simulink model "sysgenImageDoubleBuffer"  (Simulink 7.7)
settings: Solver=VariableStepDiscrete  StartTime=0.0  StopTime=((c_rx_rows_2*c_rx_cols_2)*2+(320*10))+5000  RelTol=1e-3
PreLoadFcn:
  | sysgenImageDoubleBuffer_PreLoadFcn
StartFcn:
  | tic;
undefined symbols (not defined in the file or in its folder): c_rx_cols_1, c_rx_cols_2, c_rx_rows_1, c_rx_rows_2, dpost_1, dpost_2
libraries: xbsIndex_r4 x160, dspbuff3 x6, dspsigattribs x6, dspmtrx3 x6, vipsrcs x2, simulink x2, xbsCopyrightNotice_r4 x1
(part 1 of 3)
settings Model: Creator=arvinds  LastModifiedBy=wayneh

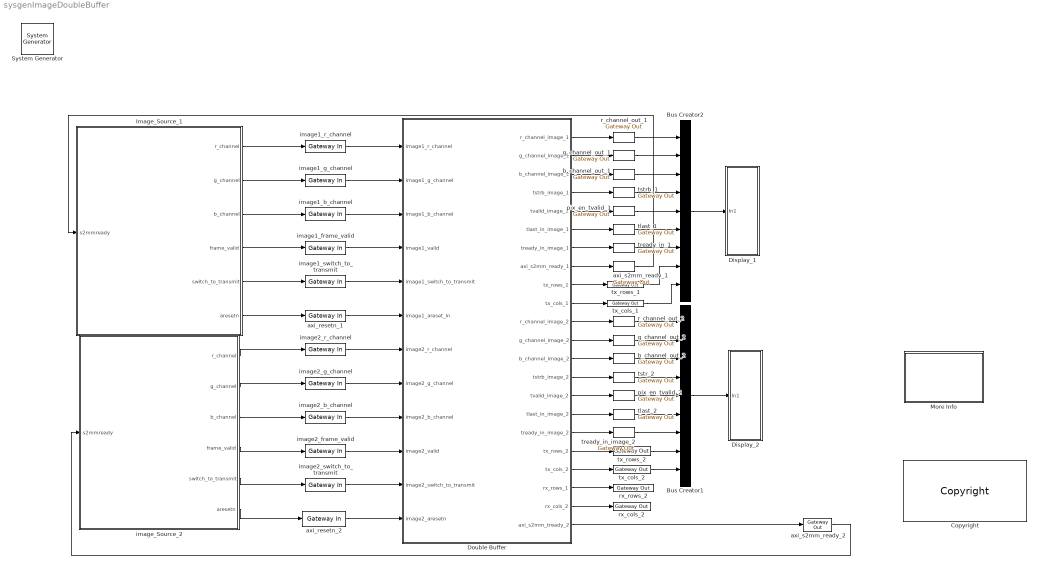
== system sysgenImageDoubleBuffer ==
  " System Generator" : xbsIndex_r4/ System Generator  Tag=genX  SystemSampleTime=-1  xilinxfamily=virtex6  part=xc6vlx240t  speed=-1  package=ff1156  synthesis_tool=XST  clock_wrapper=Clock Enables  directory=./netlist  proj_type=Project Navigator  Synth_file=XST Defaults  Impl_file=ISE Defaults  testbench=off  simulink_period=1  sysclk_period=10  dcm_input_clock_period=10  incr_netlist=off  trim_vbits=Everywhere in SubSystem  dbl_ovrd=According to Block Masks  core_generation=According to Block Masks  run_coregen=off  deprecated_control=off  eval_field=0  block_type=sysgen
      settings: block_version=12.3
  Bus Creator1 : BusCreator  Inputs=9
  Bus Creator2 : BusCreator  Inputs=9
  Copyright : xbsCopyrightNotice_r4/Copyright  copyrighttext="Copyright (c) 2011  by  Xilinx, Inc. All rights reserved.<br><br>This file contains proprietary, confidential information of Xilinx, Inc., is distributed under license from Xilinx, Inc., and may be used, copied and/or disclosed only pursuant to the terms of a valid license agreement with Xilinx, Inc. Xilinx hereby grants you a license to use this file solely for design, simulation, implementation and creation of design files limited to Xilinx devices or technologies. Use with non-Xilinx devices or technologies is expressly prohibited and immediately terminates your license unless covered by a separate agreement.<br><br>Xilinx is providing this design, code, or information \"as-is\" solely for use in developing programs and solutions for Xilinx devices, with no obligation on the part of Xilinx to provide support. By providing this design, code, or information as one possible implementation of this feature, application or standard, Xilinx is making no representation that this implementation is free from any claims of infringement. You are responsible for obtaining any rights you may require for your implementation. Xilinx expressly disclaims any warranty whatsoever with respect to the adequacy of the implementation, including but not limited to any warranties or representations that this implementation is free from claims of infringement, implied warranties of merchantability or fitness for a particular purpose.<br><br>Xilinx products are not intended for use in life support appliances, devices, or systems. Use in such applications is expressly prohibited.<br><br>Any modifications that are made to the Source Code are done at the user's sole risk and will be unsupported.<br><br>This copyright and support notice must be retained as part of this text at all times. (c) Copyright 1995-2011 Xilinx, Inc. All rights reserved."  block_type=copyright
      settings: block_version=10.1.2
      settings: infoedit=|
      | Copyright(C) 2008 by  Xilinx, Inc. All rights reserved.<br>
      | 
      | <br>
      | 
      | This file contains proprietary, confidential information of Xilinx, Inc., is distributed under license
      | 
      | from Xilinx, Inc., and may be used, copied and/or disclosed only pursuant to the terms of a valid license
      | 
      | agreement with Xilinx, Inc. Xilinx hereby grants you a license to use this file solely for design,
      | 
      | simulation, implementation and creation of design files limited to Xilinx devices or technologies. Use
      | 
      | with non-Xilinx devices or technologies is expressly prohibited and immediately terminates your license
      | 
      | unless covered by a separate agreement.<br>
      | 
      | <br>
      | 
      | Xilinx is providing this design, code, or information "as-is" solely for use in developing programs and
      | 
      | solutions for Xilinx devices, with no obligation on the part of Xilinx to provide support. By providing
      | 
      | this design, code, or information as one possible implementation of this feature, application or standard,
      | 
      | Xilinx is making no representation that this implementation is free from any claims of infringement. You
      | 
      | are responsible for obtaining any rights you may require for your implementation. Xilinx expressly disclaims
      | 
      | any warranty whatsoever with respect to the adequacy of the implementation, including but not limited to any
      | 
      | warranties or representations that this implementation is free from claims of infringement, implied warranties
      | 
      | of merchantability or fitness for a particular purpose.<br>
      | 
      | <br>
      | 
      | Xilinx products are not intended for use in life support appliances, devices, or systems. Use in such
      | 
      | applications is expressly prohibited.<br>
      | 
      | <br>
      | 
      | Any modifications that are made to the Source Code are done at the user's sole risk and will be unsupported.<br>
      | 
      | <br>
      | 
      | This copyright and support notice must be retained as part of this text at all times.
      | 
      | (c) Copyright 1995-2008 Xilinx, Inc. All rights reserved.
  Display_1 : Subsystem
  Display_2 : Subsystem
  Double Buffer : Subsystem
  Image_Source_1 : Subsystem
  More Info : Subsystem
      mask Display: disp('Double click\n for\n more information.')
  axi_resetn_1 : xbsIndex_r4/Gateway In  gui_display_data_type=Fixed-point  arith_type=Boolean  n_bits=16  bin_pt=14  preci_type=Single  exp_width=8  frac_width=24  quantization="Round  (unbiased: +/- Inf)"  overflow=Saturate  period=1  dbl_ovrd=off  timing_constraint=None  locs_specified=off  LOCs={}  inherit_from_input=off  UseAsADC=off  ADCChannel='1'  hdl_port=on  block_type=gatewayin
      settings: infoedit="Gateway in block.  Converts inputs of type Simulink integer, double and fixed point to  Xilinx fixed point type.<br><br>Hardware notes:  In hardware these blocks become top level input ports."  block_version=12.3
  axi_resetn_2 : xbsIndex_r4/Gateway In  gui_display_data_type=Fixed-point  arith_type=Boolean  n_bits=16  bin_pt=14  preci_type=Single  exp_width=8  frac_width=24  quantization="Round  (unbiased: +/- Inf)"  overflow=Saturate  period=1  dbl_ovrd=off  timing_constraint=None  locs_specified=off  LOCs={}  inherit_from_input=off  UseAsADC=off  ADCChannel='1'  hdl_port=on  block_type=gatewayin
      settings: infoedit="Gateway in block.  Converts inputs of type Simulink integer, double and fixed point to  Xilinx fixed point type.<br><br>Hardware notes:  In hardware these blocks become top level input ports."  block_version=12.3
  axi_s2mm_ready_1 : xbsIndex_r4/Gateway Out  inherit_from_input=off  hdl_port=on  timing_constraint=None  locs_specified=off  LOCs={}  UseAsDAC=off  DACChannel='1'  block_type=gatewayout
      settings: infoedit="Gateway out block.  Converts Xilinx fixed point inputs into ouputs of type Simulink integer, double, or fixed point.<br><br>Hardware notes:  In hardware these blocks become top level output ports or are discarded, depending on how they are configured."  block_version=12.3
  axi_s2mm_ready_2 : xbsIndex_r4/Gateway Out  inherit_from_input=off  hdl_port=on  timing_constraint=None  locs_specified=off  LOCs={}  UseAsDAC=off  DACChannel='1'  block_type=gatewayout
      settings: infoedit="Gateway out block.  Converts Xilinx fixed point inputs into ouputs of type Simulink integer, double, or fixed point.<br><br>Hardware notes:  In hardware these blocks become top level output ports or are discarded, depending on how they are configured."  block_version=12.3
  b_channel_out_1 : xbsIndex_r4/Gateway Out  inherit_from_input=off  hdl_port=on  timing_constraint=None  locs_specified=off  LOCs={}  UseAsDAC=off  DACChannel='1'  block_type=gatewayout
      settings: infoedit="Gateway out block.  Converts Xilinx fixed point inputs into ouputs of type Simulink integer, double, or fixed point.<br><br>Hardware notes:  In hardware these blocks become top level output ports or are discarded, depending on how they are configured."  block_version=12.3
  b_channel_out_2 : xbsIndex_r4/Gateway Out  inherit_from_input=off  hdl_port=on  timing_constraint=None  locs_specified=off  LOCs={}  UseAsDAC=off  DACChannel='1'  block_type=gatewayout
      settings: infoedit="Gateway out block.  Converts Xilinx fixed point inputs into ouputs of type Simulink integer, double, or fixed point.<br><br>Hardware notes:  In hardware these blocks become top level output ports or are discarded, depending on how they are configured."  block_version=12.3
  g_channel_out_1 : xbsIndex_r4/Gateway Out  inherit_from_input=off  hdl_port=on  timing_constraint=None  locs_specified=off  LOCs={}  UseAsDAC=off  DACChannel='1'  block_type=gatewayout
      settings: infoedit="Gateway out block.  Converts Xilinx fixed point inputs into ouputs of type Simulink integer, double, or fixed point.<br><br>Hardware notes:  In hardware these blocks become top level output ports or are discarded, depending on how they are configured."  block_version=12.3
  g_channel_out_2 : xbsIndex_r4/Gateway Out  inherit_from_input=off  hdl_port=on  timing_constraint=None  locs_specified=off  LOCs={}  UseAsDAC=off  DACChannel='1'  block_type=gatewayout
      settings: infoedit="Gateway out block.  Converts Xilinx fixed point inputs into ouputs of type Simulink integer, double, or fixed point.<br><br>Hardware notes:  In hardware these blocks become top level output ports or are discarded, depending on how they are configured."  block_version=12.3
  image1_b_channel : xbsIndex_r4/Gateway In  gui_display_data_type=Fixed-point  arith_type=Unsigned  n_bits=8  bin_pt=0  preci_type=Single  exp_width=8  frac_width=24  quantization="Round  (unbiased: +/- Inf)"  overflow=Saturate  period=1  dbl_ovrd=off  timing_constraint=None  locs_specified=off  LOCs={}  inherit_from_input=off  UseAsADC=off  ADCChannel='1'  hdl_port=on  block_type=gatewayin
      settings: infoedit="Gateway in block.  Converts inputs of type Simulink integer, double and fixed point to  Xilinx fixed point type.<br><br>Hardware notes:  In hardware these blocks become top level input ports."  block_version=12.2
  image1_frame_valid : xbsIndex_r4/Gateway In  gui_display_data_type=Fixed-point  arith_type=Boolean  n_bits=8  bin_pt=0  preci_type=Single  exp_width=8  frac_width=24  quantization="Round  (unbiased: +/- Inf)"  overflow=Saturate  period=1  dbl_ovrd=off  timing_constraint=None  locs_specified=off  LOCs={}  inherit_from_input=off  UseAsADC=off  ADCChannel='1'  hdl_port=on  block_type=gatewayin
      settings: infoedit="Gateway in block.  Converts inputs of type Simulink integer, double and fixed point to  Xilinx fixed point type.<br><br>Hardware notes:  In hardware these blocks become top level input ports."  block_version=12.2
  image1_g_channel : xbsIndex_r4/Gateway In  gui_display_data_type=Fixed-point  arith_type=Unsigned  n_bits=8  bin_pt=0  preci_type=Single  exp_width=8  frac_width=24  quantization="Round  (unbiased: +/- Inf)"  overflow=Saturate  period=1  dbl_ovrd=off  timing_constraint=None  locs_specified=off  LOCs={}  inherit_from_input=off  UseAsADC=off  ADCChannel='1'  hdl_port=on  block_type=gatewayin
      settings: infoedit="Gateway in block.  Converts inputs of type Simulink integer, double and fixed point to  Xilinx fixed point type.<br><br>Hardware notes:  In hardware these blocks become top level input ports."  block_version=12.2
  image1_r_channel : xbsIndex_r4/Gateway In  gui_display_data_type=Fixed-point  arith_type=Unsigned  n_bits=8  bin_pt=0  preci_type=Single  exp_width=8  frac_width=24  quantization="Round  (unbiased: +/- Inf)"  overflow=Saturate  period=1  dbl_ovrd=off  timing_constraint=None  locs_specified=off  LOCs={}  inherit_from_input=off  UseAsADC=off  ADCChannel='1'  hdl_port=on  block_type=gatewayin
      settings: infoedit="Gateway in block.  Converts inputs of type Simulink integer, double and fixed point to  Xilinx fixed point type.<br><br>Hardware notes:  In hardware these blocks become top level input ports."  block_version=12.2
  image1_switch_to_transmit : xbsIndex_r4/Gateway In  gui_display_data_type=Fixed-point  arith_type=Boolean  n_bits=8  bin_pt=0  preci_type=Single  exp_width=8  frac_width=24  quantization="Round  (unbiased: +/- Inf)"  overflow=Saturate  period=1  dbl_ovrd=off  timing_constraint=None  locs_specified=off  LOCs={}  inherit_from_input=off  UseAsADC=off  ADCChannel='1'  hdl_port=on  block_type=gatewayin
      settings: infoedit="Gateway in block.  Converts inputs of type Simulink integer, double and fixed point to  Xilinx fixed point type.<br><br>Hardware notes:  In hardware these blocks become top level input ports."  block_version=12.2
  image2_b_channel : xbsIndex_r4/Gateway In  gui_display_data_type=Fixed-point  arith_type=Unsigned  n_bits=8  bin_pt=0  preci_type=Single  exp_width=8  frac_width=24  quantization="Round  (unbiased: +/- Inf)"  overflow=Saturate  period=1  dbl_ovrd=off  timing_constraint=None  locs_specified=off  LOCs={}  inherit_from_input=off  UseAsADC=off  ADCChannel='1'  hdl_port=on  block_type=gatewayin
      settings: infoedit="Gateway in block.  Converts inputs of type Simulink integer, double and fixed point to  Xilinx fixed point type.<br><br>Hardware notes:  In hardware these blocks become top level input ports."  block_version=12.2
  image2_frame_valid : xbsIndex_r4/Gateway In  gui_display_data_type=Fixed-point  arith_type=Boolean  n_bits=8  bin_pt=0  preci_type=Single  exp_width=8  frac_width=24  quantization="Round  (unbiased: +/- Inf)"  overflow=Saturate  period=1  dbl_ovrd=off  timing_constraint=None  locs_specified=off  LOCs={}  inherit_from_input=off  UseAsADC=off  ADCChannel='1'  hdl_port=on  block_type=gatewayin
      settings: infoedit="Gateway in block.  Converts inputs of type Simulink integer, double and fixed point to  Xilinx fixed point type.<br><br>Hardware notes:  In hardware these blocks become top level input ports."  block_version=12.2
  image2_g_channel : xbsIndex_r4/Gateway In  gui_display_data_type=Fixed-point  arith_type=Unsigned  n_bits=8  bin_pt=0  preci_type=Single  exp_width=8  frac_width=24  quantization="Round  (unbiased: +/- Inf)"  overflow=Saturate  period=1  dbl_ovrd=off  timing_constraint=None  locs_specified=off  LOCs={}  inherit_from_input=off  UseAsADC=off  ADCChannel='1'  hdl_port=on  block_type=gatewayin
      settings: infoedit="Gateway in block.  Converts inputs of type Simulink integer, double and fixed point to  Xilinx fixed point type.<br><br>Hardware notes:  In hardware these blocks become top level input ports."  block_version=12.2
  image2_r_channel : xbsIndex_r4/Gateway In  gui_display_data_type=Fixed-point  arith_type=Unsigned  n_bits=8  bin_pt=0  preci_type=Single  exp_width=8  frac_width=24  quantization="Round  (unbiased: +/- Inf)"  overflow=Saturate  period=1  dbl_ovrd=off  timing_constraint=None  locs_specified=off  LOCs={}  inherit_from_input=off  UseAsADC=off  ADCChannel='1'  hdl_port=on  block_type=gatewayin
      settings: infoedit="Gateway in block.  Converts inputs of type Simulink integer, double and fixed point to  Xilinx fixed point type.<br><br>Hardware notes:  In hardware these blocks become top level input ports."  block_version=12.2
  image2_switch_to_transmit : xbsIndex_r4/Gateway In  gui_display_data_type=Boolean  arith_type=Boolean  n_bits=1  bin_pt=0  preci_type=Single  exp_width=8  frac_width=24  quantization="Round  (unbiased: +/- Inf)"  overflow=Saturate  period=1  dbl_ovrd=off  timing_constraint=None  locs_specified=off  LOCs={}  inherit_from_input=off  UseAsADC=off  ADCChannel='1'  hdl_port=on  block_type=gatewayin
      settings: infoedit="Gateway in block.  Converts inputs of type Simulink integer, double and fixed point to  Xilinx fixed-point or floating-point data type.<br><br>Hardware notes:  In hardware these blocks become top level input ports."  block_version=12.2
  image_Source_2 : Subsystem
  pix_en_tvalid_1 : xbsIndex_r4/Gateway Out  inherit_from_input=off  hdl_port=on  timing_constraint=None  locs_specified=off  LOCs={}  UseAsDAC=off  DACChannel='1'  block_type=gatewayout
      settings: infoedit="Gateway out block.  Converts Xilinx fixed point inputs into ouputs of type Simulink integer, double, or fixed point.<br><br>Hardware notes:  In hardware these blocks become top level output ports or are discarded, depending on how they are configured."  block_version=12.3
  pix_en_tvalid_2 : xbsIndex_r4/Gateway Out  inherit_from_input=off  hdl_port=on  timing_constraint=None  locs_specified=off  LOCs={}  UseAsDAC=off  DACChannel='1'  block_type=gatewayout
      settings: infoedit="Gateway out block.  Converts Xilinx fixed point inputs into ouputs of type Simulink integer, double, or fixed point.<br><br>Hardware notes:  In hardware these blocks become top level output ports or are discarded, depending on how they are configured."  block_version=12.3
  r_channel_out_1 : xbsIndex_r4/Gateway Out  inherit_from_input=off  hdl_port=on  timing_constraint=None  locs_specified=off  LOCs={}  UseAsDAC=off  DACChannel='1'  block_type=gatewayout
      settings: infoedit="Gateway out block.  Converts Xilinx fixed point inputs into ouputs of type Simulink integer, double, or fixed point.<br><br>Hardware notes:  In hardware these blocks become top level output ports or are discarded, depending on how they are configured."  block_version=12.3
  r_channel_out_2 : xbsIndex_r4/Gateway Out  inherit_from_input=off  hdl_port=on  timing_constraint=None  locs_specified=off  LOCs={}  UseAsDAC=off  DACChannel='1'  block_type=gatewayout
      settings: infoedit="Gateway out block.  Converts Xilinx fixed point inputs into ouputs of type Simulink integer, double, or fixed point.<br><br>Hardware notes:  In hardware these blocks become top level output ports or are discarded, depending on how they are configured."  block_version=12.3
  rx_cols_2 : xbsIndex_r4/Gateway Out  inherit_from_input=off  hdl_port=on  timing_constraint=None  locs_specified=off  LOCs={}  UseAsDAC=off  DACChannel='1'  block_type=gatewayout
      settings: infoedit="Gateway out block.  Converts Xilinx fixed point inputs into ouputs of type Simulink integer, double, or fixed point.<br><br>Hardware notes:  In hardware these blocks become top level output ports or are discarded, depending on how they are configured."  block_version=12.3
  rx_rows_2 : xbsIndex_r4/Gateway Out  inherit_from_input=off  hdl_port=on  timing_constraint=None  locs_specified=off  LOCs={}  UseAsDAC=off  DACChannel='1'  block_type=gatewayout
      settings: infoedit="Gateway out block.  Converts Xilinx fixed point inputs into ouputs of type Simulink integer, double, or fixed point.<br><br>Hardware notes:  In hardware these blocks become top level output ports or are discarded, depending on how they are configured."  block_version=12.3
  tlast_1 : xbsIndex_r4/Gateway Out  inherit_from_input=off  hdl_port=on  timing_constraint=None  locs_specified=off  LOCs={}  UseAsDAC=off  DACChannel='1'  block_type=gatewayout
      settings: infoedit="Gateway out block.  Converts Xilinx fixed point inputs into ouputs of type Simulink integer, double, or fixed point.<br><br>Hardware notes:  In hardware these blocks become top level output ports or are discarded, depending on how they are configured."  block_version=12.3
  tlast_2 : xbsIndex_r4/Gateway Out  inherit_from_input=off  hdl_port=on  timing_constraint=None  locs_specified=off  LOCs={}  UseAsDAC=off  DACChannel='1'  block_type=gatewayout
      settings: infoedit="Gateway out block.  Converts Xilinx fixed point inputs into ouputs of type Simulink integer, double, or fixed point.<br><br>Hardware notes:  In hardware these blocks become top level output ports or are discarded, depending on how they are configured."  block_version=12.3
  tready_in_1 : xbsIndex_r4/Gateway Out  inherit_from_input=off  hdl_port=on  timing_constraint=None  locs_specified=off  LOCs={}  UseAsDAC=off  DACChannel='1'  block_type=gatewayout
      settings: infoedit="Gateway out block.  Converts Xilinx fixed point inputs into ouputs of type Simulink integer, double, or fixed point.<br><br>Hardware notes:  In hardware these blocks become top level output ports or are discarded, depending on how they are configured."  block_version=12.3
  tready_in_image_2 : xbsIndex_r4/Gateway Out  inherit_from_input=off  hdl_port=on  timing_constraint=None  locs_specified=off  LOCs={}  UseAsDAC=off  DACChannel='1'  block_type=gatewayout
      settings: infoedit="Gateway out block.  Converts Xilinx fixed point inputs into ouputs of type Simulink integer, double, or fixed point.<br><br>Hardware notes:  In hardware these blocks become top level output ports or are discarded, depending on how they are configured."  block_version=12.3
  tstr_2 : xbsIndex_r4/Gateway Out  inherit_from_input=off  hdl_port=on  timing_constraint=None  locs_specified=off  LOCs={}  UseAsDAC=off  DACChannel='1'  block_type=gatewayout
      settings: infoedit="Gateway out block.  Converts Xilinx fixed point inputs into ouputs of type Simulink integer, double, or fixed point.<br><br>Hardware notes:  In hardware these blocks become top level output ports or are discarded, depending on how they are configured."  block_version=12.3
  tstrb_1 : xbsIndex_r4/Gateway Out  inherit_from_input=off  hdl_port=on  timing_constraint=None  locs_specified=off  LOCs={}  UseAsDAC=off  DACChannel='1'  block_type=gatewayout
      settings: infoedit="Gateway out block.  Converts Xilinx fixed point inputs into ouputs of type Simulink integer, double, or fixed point.<br><br>Hardware notes:  In hardware these blocks become top level output ports or are discarded, depending on how they are configured."  block_version=12.3
  tx_cols_1 : xbsIndex_r4/Gateway Out  inherit_from_input=off  hdl_port=on  timing_constraint=None  locs_specified=off  LOCs={}  UseAsDAC=off  DACChannel='1'  block_type=gatewayout
      settings: infoedit="Gateway out block.  Converts Xilinx fixed point inputs into ouputs of type Simulink integer, double, or fixed point.<br><br>Hardware notes:  In hardware these blocks become top level output ports or are discarded, depending on how they are configured."  block_version=12.3
  tx_cols_2 : xbsIndex_r4/Gateway Out  inherit_from_input=off  hdl_port=on  timing_constraint=None  locs_specified=off  LOCs={}  UseAsDAC=off  DACChannel='1'  block_type=gatewayout
      settings: infoedit="Gateway out block.  Converts Xilinx fixed point inputs into ouputs of type Simulink integer, double, or fixed point.<br><br>Hardware notes:  In hardware these blocks become top level output ports or are discarded, depending on how they are configured."  block_version=12.3
  tx_rows_1 : xbsIndex_r4/Gateway Out  inherit_from_input=off  hdl_port=on  timing_constraint=None  locs_specified=off  LOCs={}  UseAsDAC=off  DACChannel='1'  block_type=gatewayout
      settings: infoedit="Gateway out block.  Converts Xilinx fixed point inputs into ouputs of type Simulink integer, double, or fixed point.<br><br>Hardware notes:  In hardware these blocks become top level output ports or are discarded, depending on how they are configured."  block_version=12.3
  tx_rows_2 : xbsIndex_r4/Gateway Out  inherit_from_input=off  hdl_port=on  timing_constraint=None  locs_specified=off  LOCs={}  UseAsDAC=off  DACChannel='1'  block_type=gatewayout
      settings: infoedit="Gateway out block.  Converts Xilinx fixed point inputs into ouputs of type Simulink integer, double, or fixed point.<br><br>Hardware notes:  In hardware these blocks become top level output ports or are discarded, depending on how they are configured."  block_version=12.3
  wires:
  image_Source_2/4(frame_valid) -> image2_frame_valid/1
  image_Source_2/5(switch_to_transmit) -> image2_switch_to_transmit/1
  image_Source_2/6(aresetn) -> axi_resetn_2/1
  Image_Source_1/1(r_channel) -> image1_r_channel/1
  Image_Source_1/2(g_channel) -> image1_g_channel/1
  Image_Source_1/3(b_channel) -> image1_b_channel/1
  Image_Source_1/4(frame_valid) -> image1_frame_valid/1
  image_Source_2/1(r_channel) -> image2_r_channel/1
  image_Source_2/2(g_channel) -> image2_g_channel/1
  image_Source_2/3(b_channel) -> image2_b_channel/1
  Double Buffer/1(r_channel_image_1) -> r_channel_out_1/1
  Double Buffer/2(g_channel_image_1) -> g_channel_out_1/1
  Double Buffer/3(b_channel_image_1) -> b_channel_out_1/1
  Double Buffer/4(tstrb_image_1) -> tstrb_1/1
  Double Buffer/5(tvalid_image_1) -> pix_en_tvalid_1/1
  Double Buffer/6(tlast_in_image_1) -> tlast_1/1
  Double Buffer/7(tready_in_image_1) -> tready_in_1/1
  Double Buffer/8(axi_s2mm_ready_1) -> axi_s2mm_ready_1/1
  Double Buffer/9(tx_rows_1) -> tx_rows_1/1
  Double Buffer/10(tx_cols_1) -> tx_cols_1/1
  Double Buffer/11(r_channel_image_2) -> r_channel_out_2/1
  Double Buffer/12(g_channel_image_2) -> g_channel_out_2/1
  Double Buffer/13(b_channel_image_2) -> b_channel_out_2/1
  Double Buffer/14(tstrb_image_2) -> tstr_2/1
  Double Buffer/15(tvalid_image_2) -> pix_en_tvalid_2/1
  Double Buffer/16(tlast_in_image_2) -> tlast_2/1
  Double Buffer/18(tx_rows_2) -> tx_rows_2/1
  Double Buffer/19(tx_cols_2) -> tx_cols_2/1
  Double Buffer/20(rx_rows_1) -> rx_rows_2/1
  Double Buffer/21(rx_cols_2) -> rx_cols_2/1
  Double Buffer/22(axi_s2mm_tready_2) -> axi_s2mm_ready_2/1
  axi_s2mm_ready_1/1 -> Image_Source_1/1(s2mmready)
  axi_s2mm_ready_2/1 -> image_Source_2/1(s2mmready)
  Double Buffer/17(tready_in_image_2) -> tready_in_image_2/1
  image1_g_channel/1 -> Double Buffer/2(image1_g_channel)
  image1_r_channel/1 -> Double Buffer/1(image1_r_channel)
  image1_b_channel/1 -> Double Buffer/3(image1_b_channel)
  image1_frame_valid/1 -> Double Buffer/4(image1_valid)
  image1_switch_to_transmit/1 -> Double Buffer/5(image1_switch_to_transmit)
  axi_resetn_1/1 -> Double Buffer/6(image1_areset_in)
  image2_frame_valid/1 -> Double Buffer/10(image2_valid)
  image2_b_channel/1 -> Double Buffer/9(image2_b_channel)
  image2_g_channel/1 -> Double Buffer/8(image2_g_channel)
  image2_r_channel/1 -> Double Buffer/7(image2_r_channel)
  image2_switch_to_transmit/1 -> Double Buffer/11(image2_switch_to_transmit)
  axi_resetn_2/1 -> Double Buffer/12(image2_aresetn)
  r_channel_out_1/1 -> Bus Creator2/1
  g_channel_out_1/1 -> Bus Creator2/2
  b_channel_out_1/1 -> Bus Creator2/3
  tstrb_1/1 -> Bus Creator2/4
  pix_en_tvalid_1/1 -> Bus Creator2/5
  tlast_1/1 -> Bus Creator2/6
  tready_in_1/1 -> Bus Creator2/7
  tx_rows_1/1 -> Bus Creator2/8
  tx_cols_1/1 -> Bus Creator2/9
  Bus Creator2/1 -> Display_1/1(In1)
  r_channel_out_2/1 -> Bus Creator1/1
  g_channel_out_2/1 -> Bus Creator1/2
  b_channel_out_2/1 -> Bus Creator1/3
  tstr_2/1 -> Bus Creator1/4
  pix_en_tvalid_2/1 -> Bus Creator1/5
  tlast_2/1 -> Bus Creator1/6
  tready_in_image_2/1 -> Bus Creator1/7
  tx_rows_2/1 -> Bus Creator1/8
  tx_cols_2/1 -> Bus Creator1/9
  Bus Creator1/1 -> Display_2/1(In1)
  Image_Source_1/5(switch_to_transmit) -> image1_switch_to_transmit/1
  Image_Source_1/6(aresetn) -> axi_resetn_1/1

== system sysgenImageDoubleBuffer/Display_1 ==
  In1 : Inport
  Bus to Vector : BusToVector
  MATLAB Fcn : MATLABFcn  MATLABFcn=dpost_1(u(1),u(2),u(3),u(5),u(6), u(8), u(9))
  Terminator1 : Terminator
  wires:
  Bus to Vector/1 -> MATLAB Fcn/1
  MATLAB Fcn/1 -> Terminator1/1
  In1/1 -> Bus to Vector/1

== system sysgenImageDoubleBuffer/Display_2 ==
  In1 : Inport
  Bus to Vector : BusToVector
  MATLAB Fcn : MATLABFcn  MATLABFcn=dpost_2(u(1),u(2),u(3),u(5),u(6), u(8), u(9))
  Terminator1 : Terminator
  wires:
  Bus to Vector/1 -> MATLAB Fcn/1
  MATLAB Fcn/1 -> Terminator1/1
  In1/1 -> Bus to Vector/1

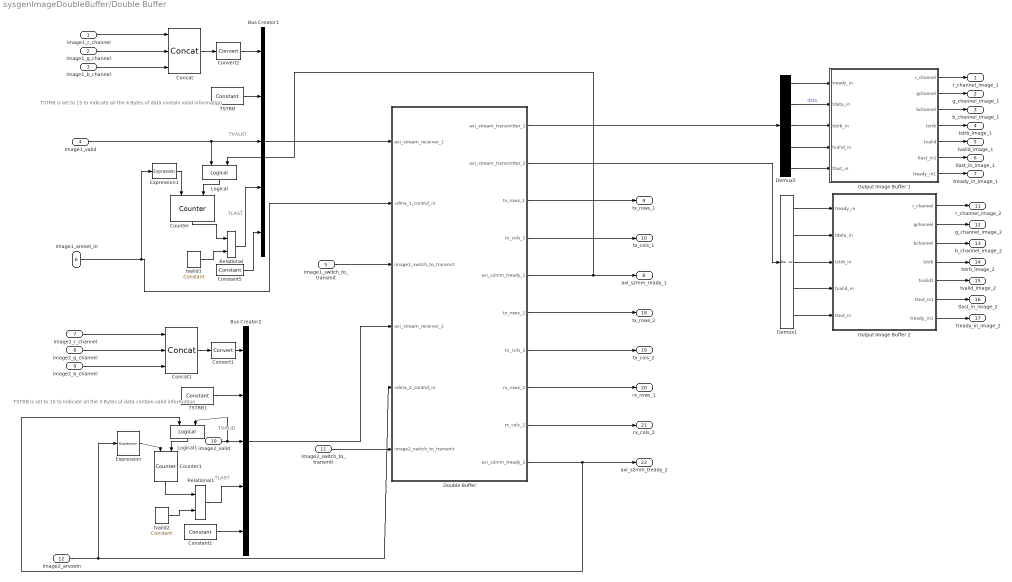
== system sysgenImageDoubleBuffer/Double Buffer ==
  note: TSTRB is set to 15 to indicate all
      | the 4 Bytes of data contain valid information
  note: TSTRB is set to 15 to indicate all
      | the 4 Bytes of data contain valid information
  note: TLAST
  note: TLAST
  note: TVALID
  note: TVALID
  image1_r_channel : Inport
  image1_g_channel : Inport  Port=2
  image1_b_channel : Inport  Port=3
  image1_valid : Inport  Port=4
  image1_switch_to_transmit : Inport  Port=5
  image1_areset_in : Inport  Port=6
  image2_r_channel : Inport  Port=7
  image2_g_channel : Inport  Port=8
  image2_b_channel : Inport  Port=9
  image2_valid : Inport  Port=10
  image2_switch_to_transmit : Inport  Port=11
  image2_aresetn : Inport  Port=12
  Bus Creator1 : BusCreator  Inputs=5
  Bus Creator2 : BusCreator  Inputs=5
  Concat : xbsIndex_r4/Concat  num_inputs=3  dbl_ovrd=off  block_type=concat
      settings: block_version=12.3
  Concat1 : xbsIndex_r4/Concat  num_inputs=3  dbl_ovrd=off  block_type=concat
      settings: block_version=12.3
  Constant1 : xbsIndex_r4/Constant  const=1  gui_display_data_type=Fixed-point  arith_type=Boolean  n_bits=16  bin_pt=14  preci_type=Single  exp_width=8  frac_width=24  explicit_period=on  period=1  equ=P=C  opselect=C  inp2=PCIN>>17  opr=+  inp1=P  carry=CIN  dbl_ovrd=off  block_type=constant
      settings: block_version=12.3
  Constant5 : xbsIndex_r4/Constant  const=1  gui_display_data_type=Fixed-point  arith_type=Boolean  n_bits=16  bin_pt=14  preci_type=Single  exp_width=8  frac_width=24  explicit_period=on  period=1  equ=P=C  opselect=C  inp2=PCIN>>17  opr=+  inp1=P  carry=CIN  dbl_ovrd=off  block_type=constant
      settings: block_version=12.3
  Convert1 : xbsIndex_r4/Convert  gui_display_data_type=Fixed-point  arith_type=Unsigned  n_bits=32  bin_pt=0  float_type=Single  exp_bits=8  fraction_bits=24  quantization=Truncate  overflow=Wrap  en=off  latency=0  dbl_ovrd=off  pipeline=off  block_type=convert
      settings: block_version=12.3
  Convert2 : xbsIndex_r4/Convert  gui_display_data_type=Fixed-point  arith_type=Unsigned  n_bits=32  bin_pt=0  float_type=Single  exp_bits=8  fraction_bits=24  quantization=Truncate  overflow=Wrap  en=off  latency=0  dbl_ovrd=off  pipeline=off  block_type=convert
      settings: block_version=12.3
  Counter : xbsIndex_r4/Counter  cnt_type=Count Limited  cnt_to=c_rx_cols_1-1  operation=Up  start_count=0  cnt_by_val=1  arith_type=Unsigned  n_bits=ceil(log2(c_rx_cols_1))+1  bin_pt=0  load_pin=off  rst=on  en=on  explicit_period=on  period=1  dbl_ovrd=off  use_behavioral_HDL=off  implementation=Fabric  block_type=counter
      settings: block_version=12.3
  Counter1 : xbsIndex_r4/Counter  cnt_type=Count Limited  cnt_to=c_rx_cols_2-1  operation=Up  start_count=0  cnt_by_val=1  arith_type=Unsigned  n_bits=ceil(log2(c_rx_cols_2))+1  bin_pt=0  load_pin=off  rst=on  en=on  explicit_period=on  period=1  dbl_ovrd=off  use_behavioral_HDL=off  implementation=Fabric  block_type=counter
      settings: block_version=12.3
  Demux1 : Demux  Outputs=5  BusSelectionMode=on
  Demux5 : Demux  Outputs=5  BusSelectionMode=on
  Double Buffer : Subsystem  mask{tx_rows_1=170, tx_cols_1=150, rx_rows_1=170, rx_cols_1=150, tx_rows_2=190, tx_cols_2=140, rx_rows_2=190, rx_cols_2=140}
  Expression : xbsIndex_r4/Expression  expression=~a  align_bp=on  en=off  latency=0  precision=Full  arith_type=Unsigned  n_bits=16  bin_pt=0  dbl_ovrd=off  block_type=expr
      settings: block_version=13.4
  Expression1 : xbsIndex_r4/Expression  expression=~a  align_bp=on  en=off  latency=0  precision=Full  arith_type=Unsigned  n_bits=16  bin_pt=0  dbl_ovrd=off  block_type=expr
      settings: block_version=13.4
  Logical : xbsIndex_r4/Logical  logical_function=AND  inputs=2  en=off  latency=0  precision=Full  arith_type=Unsigned  n_bits=16  bin_pt=0  align_bp=on  dbl_ovrd=off  block_type=logical
      settings: block_version=13.4
  Logical1 : xbsIndex_r4/Logical  logical_function=AND  inputs=2  en=off  latency=0  precision=Full  arith_type=Unsigned  n_bits=16  bin_pt=0  align_bp=on  dbl_ovrd=off  block_type=logical
      settings: block_version=13.4
  Output Image Buffer 1 : Subsystem
  Output Image Buffer 2 : Subsystem
  Relational : xbsIndex_r4/Relational  mode=a=b  en=off  latency=0  dbl_ovrd=off  block_type=relational
      settings: block_version=12.3
  Relational1 : xbsIndex_r4/Relational  mode=a=b  en=off  latency=0  dbl_ovrd=off  block_type=relational
      settings: block_version=12.3
  TSTRB : xbsIndex_r4/Constant  const=2^4-1  gui_display_data_type=Fixed-point  arith_type=Unsigned  n_bits=4  bin_pt=0  preci_type=Single  exp_width=8  frac_width=24  explicit_period=on  period=1  equ=P=C  opselect=C  inp2=PCIN>>17  opr=+  inp1=P  carry=CIN  dbl_ovrd=off  block_type=constant
      settings: block_version=12.3
  TSTRB1 : xbsIndex_r4/Constant  const=2^4-1  gui_display_data_type=Fixed-point  arith_type=Unsigned  n_bits=4  bin_pt=0  preci_type=Single  exp_width=8  frac_width=24  explicit_period=on  period=1  equ=P=C  opselect=C  inp2=PCIN>>17  opr=+  inp1=P  carry=CIN  dbl_ovrd=off  block_type=constant
      settings: block_version=12.3
  tvalid1 : xbsIndex_r4/Constant  const=c_rx_cols_1-1  gui_display_data_type=Fixed-point  arith_type=Unsigned  n_bits=ceil(log2(c_rx_cols_1+1))+1  bin_pt=0  preci_type=Single  exp_width=8  frac_width=24  explicit_period=on  period=1  equ=P=C  opselect=C  inp2=PCIN>>17  opr=+  inp1=P  carry=CIN  dbl_ovrd=off  block_type=constant
      settings: block_version=12.3
  tvalid2 : xbsIndex_r4/Constant  const=c_rx_cols_2-1  gui_display_data_type=Fixed-point  arith_type=Unsigned  n_bits=ceil(log2(c_rx_cols_2))+1  bin_pt=0  preci_type=Single  exp_width=8  frac_width=24  explicit_period=on  period=1  equ=P=C  opselect=C  inp2=PCIN>>17  opr=+  inp1=P  carry=CIN  dbl_ovrd=off  block_type=constant
      settings: block_version=12.3
  r_channel_image_1 : Outport
  g_channel_image_1 : Outport  Port=2
  b_channel_image_1 : Outport  Port=3
  tstrb_image_1 : Outport  Port=4
  tvalid_image_1 : Outport  Port=5
  tlast_in_image_1 : Outport  Port=6
  tready_in_image_1 : Outport  Port=7
  axi_s2mm_ready_1 : Outport  Port=8
  tx_rows_1 : Outport  Port=9
  tx_cols_1 : Outport  Port=10
  r_channel_image_2 : Outport  Port=11
  g_channel_image_2 : Outport  Port=12
  b_channel_image_2 : Outport  Port=13
  tstrb_image_2 : Outport  Port=14
  tvalid_image_2 : Outport  Port=15
  tlast_in_image_2 : Outport  Port=16
  tready_in_image_2 : Outport  Port=17
  tx_rows_2 : Outport  Port=18
  tx_cols_2 : Outport  Port=19
  rx_rows_1 : Outport  Port=20
  rx_cols_2 : Outport  Port=21
  axi_s2mm_tready_2 : Outport  Port=22
  wires:
  Counter/1 -> Relational/1
  tvalid1/1 -> Relational/2
  Counter1/1 -> Relational1/1
  Concat/1 -> Convert2/1
  Relational/1 -> Bus Creator1/4
  Convert2/1 -> Bus Creator1/1
  Bus Creator2/1 -> Double Buffer/4(axi_stream_receiver_2)
  TSTRB1/1 -> Bus Creator2/2
  Constant1/1 -> Bus Creator2/5
  Concat1/1 -> Convert1/1
  Convert1/1 -> Bus Creator2/1
  Bus Creator1/1 -> Double Buffer/1(axi_stream_receiver_1)
  Constant5/1 -> Bus Creator1/5
  TSTRB/1 -> Bus Creator1/2
  image1_areset_in/1 -> Double Buffer/2(vdma_1_control_in), Expression1/1
  Expression1/1 -> Counter/1
  tvalid2/1 -> Relational1/2
  image2_aresetn/1 -> Double Buffer/5(vdma_2_control_in), Expression/1
  Expression/1 -> Counter1/1
  Relational1/1 -> Bus Creator2/4
  image1_r_channel/1 -> Concat/1
  image1_g_channel/1 -> Concat/2
  image1_b_channel/1 -> Concat/3
  image1_valid/1 -> Bus Creator1/3, Logical/1
  image1_switch_to_transmit/1 -> Double Buffer/3(image1_switch_to_transmit)
  Double Buffer/1(axi_stream_transmitter_1) -> Demux5/1
  Double Buffer/2(axi_stream_transmitter_2) -> Demux1/1
  Double Buffer/3(tx_rows_1) -> tx_rows_1/1
  Double Buffer/4(tx_cols_1) -> tx_cols_1/1
  image2_r_channel/1 -> Concat1/1
  image2_g_channel/1 -> Concat1/2
  image2_b_channel/1 -> Concat1/3
  Double Buffer/5(axi_s2mm_tready_1) -> axi_s2mm_ready_1/1, Logical/2
  Double Buffer/6(tx_rows_2) -> tx_rows_2/1
  image2_valid/1 -> Bus Creator2/3, Logical1/2
  Double Buffer/7(tx_cols_2) -> tx_cols_2/1
  Double Buffer/8(rx_rows_2) -> rx_rows_1/1
  Double Buffer/9(rx_cols_2) -> rx_cols_2/1
  Double Buffer/10(axi_s2mm_tready_2) -> axi_s2mm_tready_2/1, Logical1/1
  image2_switch_to_transmit/1 -> Double Buffer/6(image2_switch_to_transmit)
  Demux5/1 -> Output Image Buffer 1/1(tready_in)
  Demux5/2 -> Output Image Buffer 1/2(tdata_in)  "data"
  Demux5/4 -> Output Image Buffer 1/4(tvalid_in)
  Demux5/5 -> Output Image Buffer 1/5(tlast_in)
  Demux5/3 -> Output Image Buffer 1/3(tstrb_in)
  Output Image Buffer 1/1(r_channel) -> r_channel_image_1/1
  Output Image Buffer 1/2(gchannel) -> g_channel_image_1/1
  Output Image Buffer 1/3(bchannel) -> b_channel_image_1/1
  Output Image Buffer 1/4(tstrb) -> tstrb_image_1/1
  Output Image Buffer 1/5(tvalid) -> tvalid_image_1/1
  Output Image Buffer 1/6(tlast_in1) -> tlast_in_image_1/1
  Output Image Buffer 1/7(tready_in1) -> tready_in_image_1/1
  Demux1/1 -> Output Image Buffer 2/1(tready_in)
  Demux1/2 -> Output Image Buffer 2/2(tdata_in)
  Demux1/4 -> Output Image Buffer 2/4(tvalid_in)
  Demux1/5 -> Output Image Buffer 2/5(tlast_in)
  Demux1/3 -> Output Image Buffer 2/3(tstrb_in)
  Output Image Buffer 2/1(r_channel) -> r_channel_image_2/1
  Output Image Buffer 2/2(gchannel) -> g_channel_image_2/1
  Output Image Buffer 2/3(bchannel) -> b_channel_image_2/1
  Output Image Buffer 2/4(tstrb) -> tstrb_image_2/1
  Output Image Buffer 2/5(tvalid1) -> tvalid_image_2/1
  Output Image Buffer 2/6(tlast_in1) -> tlast_in_image_2/1
  Output Image Buffer 2/7(tready_in1) -> tready_in_image_2/1
  Logical/1 -> Counter/2
  Logical1/1 -> Counter1/2

== system sysgenImageDoubleBuffer/Image_Source_1 ==
  note: Image source is read from Disk and supplied to the AXI Stream Slave Ports of the VDMA Interface 4.0 .
      | 16 lines of the image constitue a frame and the TLAST signifies the end of each frame. Each RGB
      | pixel is concatenated and packed into a 32 bit word and passed to the VDMA. TSTRB for each word
      | is set to 0xF to indicate all 4 byte lines of the input data are valid.
  s2mmready : Inport
  Image_source_1 : Subsystem
  Step1 : Step  Time=32  SampleTime=1
  Subsystem1 : Subsystem
  r_channel : Outport
  g_channel : Outport  Port=2
  b_channel : Outport  Port=3
  frame_valid : Outport  Port=4
  switch_to_transmit : Outport  Port=5
  aresetn : Outport  Port=6
  wires:
  Image_source_1/1(r_channel) -> r_channel/1
  Image_source_1/2(g_channel) -> g_channel/1
  Image_source_1/3(b_channel) -> b_channel/1
  Step1/1 -> Subsystem1/2(aresetn), aresetn/1
  Subsystem1/2(valid_pop) -> Image_source_1/2(valid_pop), frame_valid/1
  Subsystem1/3(transmit_image_1) -> switch_to_transmit/1
  s2mmready/1 -> Subsystem1/1(ready)
  Subsystem1/1(valid_push) -> Image_source_1/1(valid_push)

== system sysgenImageDoubleBuffer/More Info ==
  note: This design shows how to create a generic double data buffer using SysGen External Memory Interface simulation model block based
      | on the VDMA IP behaviour. The design behaves similarly to a Dual Port RAM with two read , write data ports and some simple control
      | I/O ports.
      |
      | For this particular configuration, each buffer reads a complete frame of an input image file and stores it in the VDMA system memory.
      | The same image is then transmitted via axi_stream_transmitter ports. At the top-level, the parameters are provided so you can configure
      | the design to read and write different size of 2D images.
      |
      | Block Descriptors:
      |
      | The VDMA can be configured to transfer multiple frames of data where each frame is a 2D data characterized by :
      | START_ADDRESS : The Physical location in memory where the first Byte of the frame is read from or written to.
      | HSIZE : Number of horizontal bytes
      | VSIZE : Number of vertical lines of transfer
      | STRIDE : The address offset between the start byte in each line.
      |
      | In this design, users can manipulate how and when to read the image stored in the VDMA system memory by modifying these two M-code files:
      |    -  xldScatterGatherEngineBlockTransfer_1.m for the first buffer channel
      |    -  xldScatterGatherEngineBlockTransfer_2.m for the second buffer channel
      | For example, to read from the first buffer , the START_ADDRESS will need to be set to zero. On the other hand, to read from the second buffer,
      | the START_ADDRESS will need need to be offset  by the size of the first input image.
      |
      | Both buffers share the same M-code file (xlWriteControlRegister_db.m) to control data and address registers of the AXI VDMA operation.
  note: Double Buffer Demo

== system sysgenImageDoubleBuffer/image_Source_2 ==
  note: Image source is read from Disk and supplied to the AXI Stream Slave Ports of the VDMA Interface 4.0 .
      | 16 lines of the image constitue a frame and the TLAST signifies the end of each frame. Each RGB
      | pixel is concatenated and packed into a 32 bit word and passed to the VDMA. TSTRB for each word
      | is set to 0xF to indicate all 4 byte lines of the input data are valid.
  s2mmready : Inport
  Step4 : Step  Time=32  SampleTime=1
  Subsystem : Subsystem
  image_source_2 : Subsystem
  r_channel : Outport
  g_channel : Outport  Port=2
  b_channel : Outport  Port=3
  frame_valid : Outport  Port=4
  switch_to_transmit : Outport  Port=5
  aresetn : Outport  Port=6
  wires:
  Step4/1 -> Subsystem/2(aresetn), aresetn/1
  Subsystem/2(valid_pop) -> image_source_2/2(valid_pop), frame_valid/1
  image_source_2/1(r_channel) -> r_channel/1
  image_source_2/2(g_channel) -> g_channel/1
  image_source_2/3(b_channel) -> b_channel/1
  Subsystem/3(transmit_image_2) -> switch_to_transmit/1
  s2mmready/1 -> Subsystem/1(ready)
  Subsystem/1(valid_push) -> image_source_2/1(valid_push)

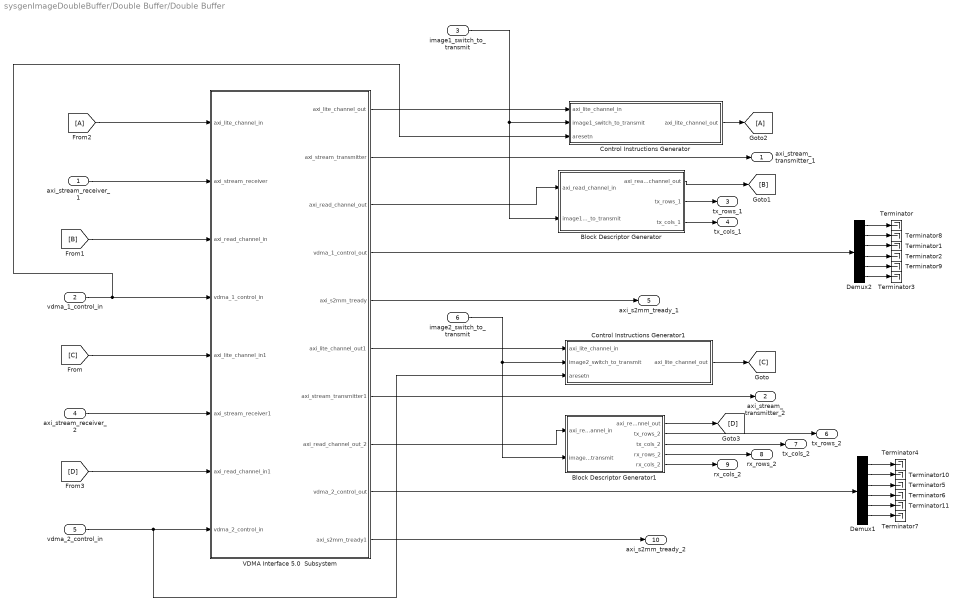
== system sysgenImageDoubleBuffer/Double Buffer/Double Buffer ==
  axi_stream_receiver_1 : Inport
  vdma_1_control_in : Inport  Port=2
  image1_switch_to_transmit : Inport  Port=3
  axi_stream_receiver_2 : Inport  Port=4
  vdma_2_control_in : Inport  Port=5
  image2_switch_to_transmit : Inport  Port=6
  Block Descriptor Generator : Subsystem  mask{tx_rows_1=tx_rows_1, tx_cols_1=tx_cols_1, rx_rows_1=rx_rows_1, rx_cols_1=rx_cols_1}
  Block Descriptor Generator1 : Subsystem  mask{tx_rows_2=tx_rows_2, tx_cols_2=tx_cols_2, rx_rows_2=rx_rows_2, rx_cols_2=rx_cols_2}
  Control Instructions Generator : Subsystem
  Control Instructions Generator1 : Subsystem
  Demux1 : Demux  Outputs=6  BusSelectionMode=on
  Demux2 : Demux  Outputs=6  BusSelectionMode=on
  Terminator{,1..11} (12 alike) : Terminator
  VDMA Interface 5.0  Subsystem : Subsystem
  axi_stream_transmitter_1 : Outport
  axi_stream_transmitter_2 : Outport  Port=2
  tx_rows_1 : Outport  Port=3
  tx_cols_1 : Outport  Port=4
  axi_s2mm_tready_1 : Outport  Port=5
  tx_rows_2 : Outport  Port=6
  tx_cols_2 : Outport  Port=7
  rx_rows_2 : Outport  Port=8
  rx_cols_2 : Outport  Port=9
  axi_s2mm_tready_2 : Outport  Port=10
  wires:
  VDMA Interface 5.0  Subsystem/1(axi_lite_channel_out) -> Control Instructions Generator/1(axi_lite_channel_in)
  VDMA Interface 5.0  Subsystem/3(axi_read_channel_out) -> Block Descriptor Generator/1(axi_read_channel_in)
  VDMA Interface 5.0  Subsystem/8(axi_read_channel_out_2) -> Block Descriptor Generator1/1(axi_read_channel_in)
  Control Instructions Generator1/1(axi_lite_channel_out) -> [C]
  [C] -> VDMA Interface 5.0  Subsystem/5(axi_lite_channel_in1)
  Block Descriptor Generator/1(axi_read_channel_out) -> [B]
  [B] -> VDMA Interface 5.0  Subsystem/3(axi_read_channel_in)
  Control Instructions Generator/1(axi_lite_channel_out) -> [A]
  [A] -> VDMA Interface 5.0  Subsystem/1(axi_lite_channel_in)
  Block Descriptor Generator1/1(axi_read_channel_out) -> [D]
  [D] -> VDMA Interface 5.0  Subsystem/7(axi_read_channel_in1)
  VDMA Interface 5.0  Subsystem/6(axi_lite_channel_out1) -> Control Instructions Generator1/1(axi_lite_channel_in)
  vdma_2_control_in/1 -> VDMA Interface 5.0  Subsystem/8(vdma_2_control_in), Control Instructions Generator1/3(aresetn)
  vdma_1_control_in/1 -> VDMA Interface 5.0  Subsystem/4(vdma_1_control_in), Control Instructions Generator/3(aresetn)
  axi_stream_receiver_1/1 -> VDMA Interface 5.0  Subsystem/2(axi_stream_receiver)
  axi_stream_receiver_2/1 -> VDMA Interface 5.0  Subsystem/6(axi_stream_receiver1)
  VDMA Interface 5.0  Subsystem/2(axi_stream_transmitter) -> axi_stream_transmitter_1/1
  VDMA Interface 5.0  Subsystem/7(axi_stream_transmitter1) -> axi_stream_transmitter_2/1
  VDMA Interface 5.0  Subsystem/9(vdma_2_control_out) -> Demux1/1
  Demux1/2 -> Terminator10/1
  Demux1/5 -> Terminator11/1
  VDMA Interface 5.0  Subsystem/4(vdma_1_control_out) -> Demux2/1
  Demux2/1 -> Terminator/1
  Demux2/3 -> Terminator1/1
  Demux2/4 -> Terminator2/1
  Demux2/6 -> Terminator3/1
  Demux1/1 -> Terminator4/1
  Demux1/3 -> Terminator5/1
  Demux1/4 -> Terminator6/1
  Demux1/6 -> Terminator7/1
  Demux2/2 -> Terminator8/1
  Demux2/5 -> Terminator9/1
  Block Descriptor Generator1/2(tx_rows_2) -> tx_rows_2/1
  Block Descriptor Generator1/3(tx_cols_2) -> tx_cols_2/1
  Block Descriptor Generator1/4(rx_rows_2) -> rx_rows_2/1
  Block Descriptor Generator1/5(rx_cols_2) -> rx_cols_2/1
  Block Descriptor Generator/2(tx_rows_1) -> tx_rows_1/1
  Block Descriptor Generator/3(tx_cols_1) -> tx_cols_1/1
  VDMA Interface 5.0  Subsystem/5(axi_s2mm_tready) -> axi_s2mm_tready_1/1
  VDMA Interface 5.0  Subsystem/10(axi_s2mm_tready1) -> axi_s2mm_tready_2/1
  image1_switch_to_transmit/1 -> Block Descriptor Generator/2(image1_switch_to_transmit), Control Instructions Generator/2(image1_switch_to_transmit)
  image2_switch_to_transmit/1 -> Block Descriptor Generator1/2(image2_switch_to_transmit), Control Instructions Generator1/2(image2_switch_to_transmit)

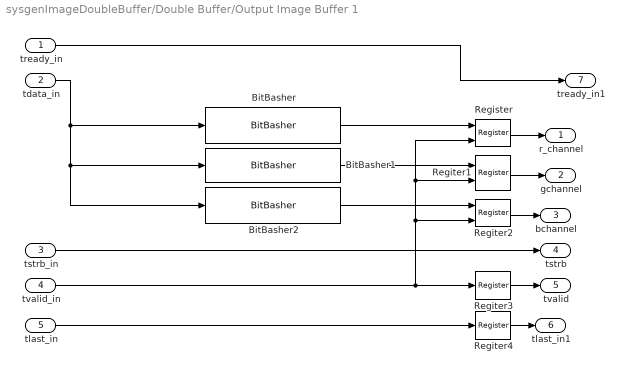
== system sysgenImageDoubleBuffer/Double Buffer/Output Image Buffer 1 ==
  tready_in : Inport
  tdata_in : Inport  Port=2
  tstrb_in : Inport  Port=3
  tvalid_in : Inport  Port=4
  tlast_in : Inport  Port=5
  BitBasher : xbsIndex_r4/BitBasher  bitexpr=|  display_expr=off  sr_1=1  arith_type1=Unsigned  bin_pt1=0  sr_2=2  arith_type2=Unsigned  bin_pt2=0  sr_3=3  arith_type3=Unsigned  bin_pt3=0  sr_4=4  arith_type4=Unsigned  bin_pt4=0  dbl_ovrd=off  block_type=bitbasher
      | <!DOCTYPE HTML PUBLIC "-//W3C//DTD HTML 4.0//EN" "http://www.w3.org/TR/REC-html40/strict.dtd">
      | <html><head><meta name="qrichtext" content="1" /><style type="text/css">
      | p, li { white-space: pre-wrap; }
      | </style></head><body style=" font-family:'MS Shell Dlg 2'; font-size:7.8pt; font-weight:400; font-style:normal;">
      | <p style=" margin-top:12px; margin-bottom:12px; margin-left:0px; margin-right:0px; -qt-block-indent:0; text-indent:0px;"><span style=" font-family:'MS Shell Dlg'; font-size:8pt;">r_channel={mem[23:16]}</span></p></body></html>
      settings: block_version=12.3
  BitBasher1 : xbsIndex_r4/BitBasher  bitexpr=|  display_expr=off  sr_1=1  arith_type1=Unsigned  bin_pt1=0  sr_2=2  arith_type2=Unsigned  bin_pt2=0  sr_3=3  arith_type3=Unsigned  bin_pt3=0  sr_4=4  arith_type4=Unsigned  bin_pt4=0  dbl_ovrd=off  block_type=bitbasher
      | <!DOCTYPE HTML PUBLIC "-//W3C//DTD HTML 4.0//EN" "http://www.w3.org/TR/REC-html40/strict.dtd">
      | <html><head><meta name="qrichtext" content="1" /><style type="text/css">
      | p, li { white-space: pre-wrap; }
      | </style></head><body style=" font-family:'MS Shell Dlg 2'; font-size:7.8pt; font-weight:400; font-style:normal;">
      | <p style=" margin-top:12px; margin-bottom:12px; margin-left:0px; margin-right:0px; -qt-block-indent:0; text-indent:0px;"><span style=" font-family:'MS Shell Dlg'; font-size:8pt;">g_channel={mem[15:8]}</span></p></body></html>
      settings: block_version=12.3
  BitBasher2 : xbsIndex_r4/BitBasher  bitexpr=|  display_expr=off  sr_1=1  arith_type1=Unsigned  bin_pt1=0  sr_2=2  arith_type2=Unsigned  bin_pt2=0  sr_3=3  arith_type3=Unsigned  bin_pt3=0  sr_4=4  arith_type4=Unsigned  bin_pt4=0  dbl_ovrd=off  block_type=bitbasher
      | <!DOCTYPE HTML PUBLIC "-//W3C//DTD HTML 4.0//EN" "http://www.w3.org/TR/REC-html40/strict.dtd">
      | <html><head><meta name="qrichtext" content="1" /><style type="text/css">
      | p, li { white-space: pre-wrap; }
      | </style></head><body style=" font-family:'MS Shell Dlg 2'; font-size:7.8pt; font-weight:400; font-style:normal;">
      | <p style=" margin-top:12px; margin-bottom:12px; margin-left:0px; margin-right:0px; -qt-block-indent:0; text-indent:0px;"><span style=" font-family:'MS Shell Dlg'; font-size:8pt;">b_channel={mem[7:0]}</span></p></body></html>
      settings: block_version=12.3
  Register : xbsIndex_r4/Register  init=0  rst=off  en=on  dbl_ovrd=off  block_type=register
      settings: block_version=12.3
  Regiter1 : xbsIndex_r4/Register  init=0  rst=off  en=on  dbl_ovrd=off  block_type=register
      settings: block_version=12.3
  Regiter2 : xbsIndex_r4/Register  init=0  rst=off  en=on  dbl_ovrd=off  block_type=register
      settings: block_version=12.3
  Regiter3 : xbsIndex_r4/Register  init=0  rst=off  en=off  dbl_ovrd=off  block_type=register
      settings: block_version=12.3
  Regiter4 : xbsIndex_r4/Register  init=0  rst=off  en=off  dbl_ovrd=off  block_type=register
      settings: block_version=12.3
  r_channel : Outport
  gchannel : Outport  Port=2
  bchannel : Outport  Port=3
  tstrb : Outport  Port=4
  tvalid : Outport  Port=5
  tlast_in1 : Outport  Port=6
  tready_in1 : Outport  Port=7
  wires:
  tready_in/1 -> tready_in1/1
  tvalid_in/1 -> Regiter2/2, Regiter1/2, Register/2, Regiter3/1
  tdata_in/1 -> BitBasher2/1, BitBasher1/1, BitBasher/1
  BitBasher/1 -> Register/1
  BitBasher1/1 -> Regiter1/1
  BitBasher2/1 -> Regiter2/1
  Register/1 -> r_channel/1
  Regiter1/1 -> gchannel/1
  Regiter2/1 -> bchannel/1
  Regiter3/1 -> tvalid/1
  tlast_in/1 -> Regiter4/1
  Regiter4/1 -> tlast_in1/1
  tstrb_in/1 -> tstrb/1
